simulink model "TSR_System"  (Simulink 7.8)
settings: Solver=ode5  StartTime=0.0  StopTime=inf  FixedStep=1/100  RelTol=1e-3
undefined symbols (not defined in the file): gray, Rec, SDTV
libraries: simulink x4, visionanalysis x2, visiontextngfix x2, visionsinks x2, visionconversions x1, visionstatistics x1
settings Model: Creator=Krzysztof  LastModifiedBy=MarcinB
settings OptimizationCC: InlineParams=on
settings DebuggingCC: SolverPrmCheckMsg=none  MultiTaskCondExecSysMsg=none  MultiTaskRateTransMsg=warning  FcnCallInpInsideContextMsg=Use local settings
settings SFSimCC: SimParseCustomCode=off

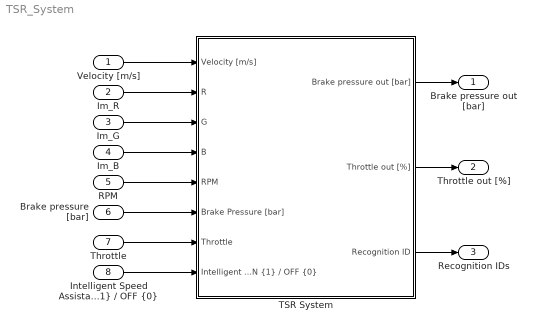
== system TSR_System ==
  Velocity [m/s] : Inport  Interpolate=off
  Im_R : Inport  Port=2
  Im_G : Inport  Port=3
  Im_B : Inport  Port=4
  RPM : Inport  Port=5
  Brake pressure [bar] : Inport  Port=6
  Throttle : Inport  Port=7
  "Intelligent Speed Assistance ON {1} / OFF {0}" : Inport  Port=8
  TSR System : Subsystem  mask{exp_freq=25, dfreq=50, GUI_freq=25, ImgRes=[600 800], DetectionTreshholdValue=0.75, RecognitionTreshholdValue=0.75, NumLimit=5, cdt=3, gdt=5, Tblink=0.5, MaxBrakePressure=150, Perc=20}
      mask prompts: exp_freq "Experiments frequency [Hz]"; dfreq "System frequency [Hz]"; GUI_freq "GUI display frequency [Hz]"; ImgRes "Image resolution"; DetectionTreshholdValue "Detection treshhold value"; RecognitionTreshholdValue "Recognition treshhold value"; NumLimit "Maximum number of objects to extract from image"; cdt "Holding time of recognized sign (colour) [s]"; gdt "Holding time of recognized sign (gray) [s]"; Tblink "Speed limit warning - blinking period [s]"; MaxBrakePressure "Maximum braking pressure [bar]"; Perc "Maximum applicable percentage of deceleration by ISA [%]"
      mask init:
      | %% Generate templates (mat files) if missing
      | if ~exist('DetectTemplates.mat','file')
      |     detection_templates;
      | end
      | if ~exist('RecognitionTemplates.mat','file')
      |     recognition_templates;
      | end
      | 
      | % Load templates into workspace
      | load DetectTemplates.mat
      | load RecognitionTemplates.mat
      | 
      | % Number of templates
      | NoD = size(DetectTemplates,2);
      | NoR = size(RecognitionTemplates,2);
  Brake pressure out [bar] : Outport
  Throttle out [%] : Outport  Port=2
  Recognition IDs : Outport  Port=3
  wires:
  Im_R/1 -> TSR System/2(R)
  Im_G/1 -> TSR System/3(G)
  Im_B/1 -> TSR System/4(B)
  Velocity [m/s]/1 -> TSR System/1(Velocity [m/s])
  Brake pressure [bar]/1 -> TSR System/6(Brake Pressure [bar])
  RPM/1 -> TSR System/5(RPM)
  TSR System/1(Brake pressure out [bar]) -> Brake pressure out [bar]/1
  "Intelligent Speed Assistance ON {1} / OFF {0}"/1 -> TSR System/8("Intelligent Speed Assistance ON {1} / OFF {0}")
  Throttle/1 -> TSR System/7(Throttle)
  TSR System/2("Throttle out [%] ") -> Throttle out [%]/1
  TSR System/3(Recognition ID) -> Recognition IDs/1

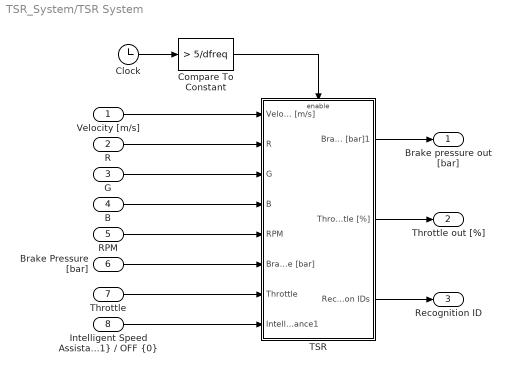
== system TSR_System/TSR System ==
  Velocity [m/s] : Inport  SampleTime=[0 0]
  R : Inport  Port=2  OutDataTypeStr=uint8  PortDimensions=ImgRes
  G : Inport  Port=3  OutDataTypeStr=uint8  PortDimensions=ImgRes
  B : Inport  Port=4  OutDataTypeStr=uint8  PortDimensions=ImgRes
  RPM : Inport  Port=5  SampleTime=[0 0]
  Brake Pressure [bar] : Inport  Port=6  SampleTime=[0 0]
  Throttle : Inport  Port=7
  "Intelligent Speed Assistance ON {1} / OFF {0}" : Inport  Port=8
  Clock : Clock
  Compare To Constant : simulink/Logic and Bit Operations/Compare To Constant  relop=>  const=5/dfreq  OutDataTypeStr=boolean
  TSR : Subsystem
  Brake pressure out [bar] : Outport
  "Throttle out [%] " : Outport  Port=2
  Recognition ID : Outport  Port=3
  wires:
  Clock/1 -> Compare To Constant/1
  Compare To Constant/1 -> TSR/Enable
  TSR/1(Braking pressure [bar]1) -> Brake pressure out [bar]/1
  TSR/2(Throttle [%]) -> "Throttle out [%] "/1
  TSR/3(Recognition IDs) -> Recognition ID/1
  Velocity [m/s]/1 -> TSR/1(Velocity [m/s])
  R/1 -> TSR/2(R)
  G/1 -> TSR/3(G)
  B/1 -> TSR/4(B)
  RPM/1 -> TSR/5(RPM)
  Throttle/1 -> TSR/7(Throttle)
  "Intelligent Speed Assistance ON {1} / OFF {0}"/1 -> TSR/8(Intelligent Speed Assistance1)
  Brake Pressure [bar]/1 -> TSR/6(Brake Pressure [bar])

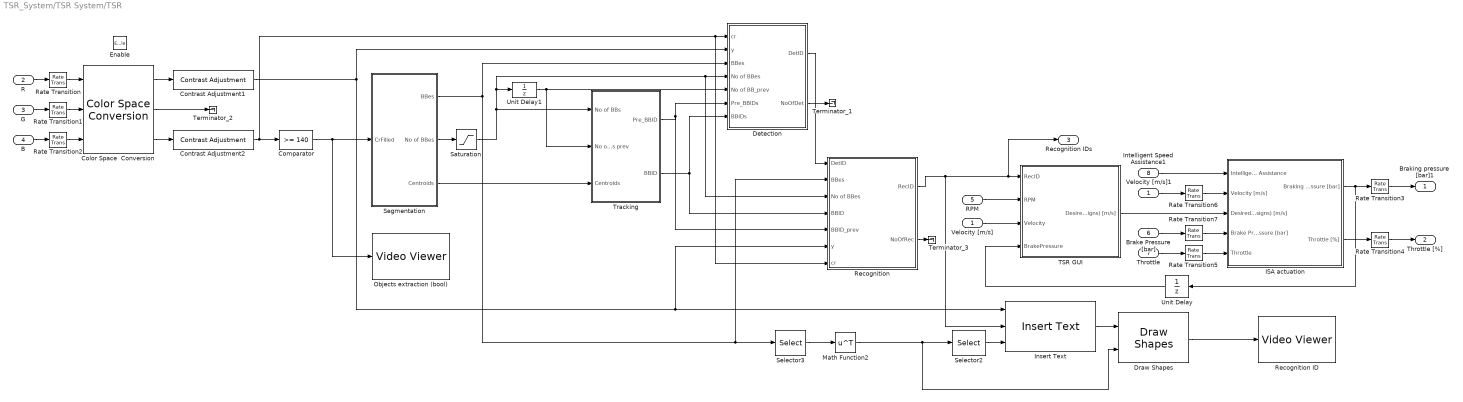
== system TSR_System/TSR System/TSR ==
  Velocity [m/s] : Inport  SampleTime=[0 0]
  R : Inport  Port=2  OutDataTypeStr=uint8  PortDimensions=ImgRes
  G : Inport  Port=3
  B : Inport  Port=4  OutDataTypeStr=uint8  PortDimensions=ImgRes
  RPM : Inport  Port=5  SampleTime=[0 0]
  Brake Pressure [bar] : Inport  Port=6  SampleTime=[0 0]
  Throttle : Inport  Port=7  SampleTime=0
  Intelligent Speed Assistance1 : Inport  Port=8
  Enable : EnablePort
  Color Space  Conversion : visionconversions/Color Space  Conversion  conversion=Obsolete  conversionActive=R'G'B' to Y'CbCr  wp_str=D65  rec=Rec. 601 (SDTV)  sys=1125/60/2:1  imagePorts=Separate color signals
  Comparator : simulink/Logic and Bit Operations/Compare To Constant  relop=>=  const=140  OutDataTypeStr=boolean
  Contrast Adjustment1 : visionanalysis/Contrast Adjustment  methodInputRange=Full input data range [min max]  rangeIn=[0 255]  fracSaturate=[1 1]  isBinNum=on  binNum=256  methodOutputRange=Full data type range  rangeOut=[0 255]  prod1Mode=Binary point scaling  prod1WordLength=32  prod1FracLength=16  prod2Mode=Binary point scaling  prod2WordLength=32  prod2FracLength=16  roundingMode=Floor  overflowMode=off
  Contrast Adjustment2 : visionanalysis/Contrast Adjustment  methodInputRange=Full input data range [min max]  rangeIn=[0 255]  fracSaturate=[1 1]  isBinNum=on  binNum=256  methodOutputRange=Full data type range  rangeOut=[0 255]  prod1Mode=Binary point scaling  prod1WordLength=32  prod1FracLength=16  prod2Mode=Binary point scaling  prod2WordLength=32  prod2FracLength=16  roundingMode=Floor  overflowMode=off
  Detection : Subsystem
  Draw Shapes : visiontextngfix/Draw Shapes  shape=Rectangles  fill=off  fillClrSource=Specify via dialog  display=White  intensity=200  color=[200 255 100]  opacity=0.6  viewport=Entire image  antialiasing=off  inType=Obsolete  imagePorts=One multidimensional signal  prodOutputMode=Binary point scaling  prodOutputWordLength=32  prodOutputFracLength=14  memoryMode=Specify word length  memoryWordLength=16  memoryFracLength=15  roundingMode=Floor  overflowMode=off
  ISA actuation : Subsystem
  Insert Text : visiontextngfix/Insert Text  inputType=Obsolete  theText='%d'  fontFace=LucidaSansRegular  dummyVar1=0  blockFontSize=12  antiAliased=on  getTextLocFrom=Input port  textLoc=[1 1]  getTextColorFrom=Specify via dialog  textColor=255*ones(1,NumLimit);  getTextIntensityFrom=Specify via dialog  textIntensity=0  getTextOpacityFrom=Specify via dialog  textOpacity=1.0  dummyVar2=0  dummyVar3=0  dummyVar4=0  imagePorts=One multidimensional signal  isInputTransposed=off
  Math Function2 : Math  Operator=transpose  SaturateOnIntegerOverflow=on
  Objects extraction (bool) : visionsinks/Video Viewer  inputType=Obsolete7b  imagePorts=One multidimensional signal  useColorMap=off  colormapValue=gray(256)  specRange=off  minInputVal=0  maxInputVal=255  FigPos=[1027 701 606 494]  AxisZoom=on  trueSizedOnce=off  OpenAtMdlStart=on
  Rate Transition : RateTransition  Integrity=off  OutPortSampleTime=1/dfreq
  Rate Transition1 : RateTransition  Integrity=off  OutPortSampleTime=1/dfreq
  Rate Transition2 : RateTransition  Integrity=off  OutPortSampleTime=1/dfreq
  Rate Transition3 : RateTransition  Integrity=off  OutPortSampleTime=0
  Rate Transition4 : RateTransition  Integrity=off  OutPortSampleTime=0
  Rate Transition5 : RateTransition  Integrity=off  OutPortSampleTime=1/GUI_freq
  Rate Transition6 : RateTransition  Integrity=off  OutPortSampleTime=1/GUI_freq
  Rate Transition7 : RateTransition  Integrity=off  OutPortSampleTime=1/GUI_freq
  Recognition : Subsystem
  Recognition ID : visionsinks/Video Viewer  inputType=Obsolete7b  imagePorts=One multidimensional signal  useColorMap=off  colormapValue=gray(256)  specRange=off  minInputVal=0  maxInputVal=255  FigPos=[130 747 808 632]  AxisZoom=on  trueSizedOnce=off  OpenAtMdlStart=on
  Saturation : Saturate  UpperLimit=NumLimit  LowerLimit=0
  Segmentation : Subsystem
  Selector2 : Selector  NumberOfDimensions=2  InputPortWidth=3  IndexOptions=Select all,Index vector (dialog)  Indices=[1 2],[1, 2]  OutputSizes=1,1
  Selector3 : Selector  NumberOfDimensions=2  InputPortWidth=3  IndexOptions=Index vector (dialog),Select all  Indices=[2, 1, 4, 3],1  OutputSizes=1,1
  TSR GUI : Subsystem
  Terminator_1 : Terminator
  Terminator_2 : Terminator
  Terminator_3 : Terminator
  Tracking : Subsystem
  Unit Delay : UnitDelay  SampleTime=-1
  Unit Delay1 : UnitDelay  SampleTime=-1
  Velocity [m/s]1 : InportShadow  Port=1  SampleTime=[0 0]
  Braking pressure [bar]1 : Outport
  Throttle [%] : Outport  Port=2
  Recognition IDs : Outport  Port=3  SampleTime=1/dfreq
  wires:
  Color Space  Conversion/3 -> Contrast Adjustment2/1
  Color Space  Conversion/1 -> Contrast Adjustment1/1
  Color Space  Conversion/2 -> Terminator_2/1
  Segmentation/1(BBes) -> Detection/3(BBes), Recognition/2(BBes), Selector3/1
  Segmentation/2(No of BBes) -> Saturation/1
  Contrast Adjustment2/1 -> Comparator/1, Detection/1(cr), Recognition/7(cr)
  Segmentation/3(Centroids) -> Tracking/3(Centroids)
  Tracking/2(BBID) -> Detection/7(BBIDs), Recognition/4(BBID)
  Tracking/1(Pre_BBID) -> Detection/6(Pre_BBIDs), Recognition/5(BBID_prev)
  Contrast Adjustment1/1 -> Detection/2(y), Recognition/6(y), Insert Text/1
  Unit Delay1/1 -> Tracking/2(No of BBs prev), Detection/5(No of BB_prev)
  Recognition/1(RecID) -> TSR GUI/1(RecID), Recognition IDs/1, Insert Text/2
  R/1 -> Rate Transition/1
  G/1 -> Rate Transition1/1
  B/1 -> Rate Transition2/1
  Rate Transition/1 -> Color Space  Conversion/1
  Rate Transition1/1 -> Color Space  Conversion/2
  Rate Transition2/1 -> Color Space  Conversion/3
  Saturation/1 -> Unit Delay1/1, Detection/4(No of BBes), Recognition/3(No of BBes), Tracking/1(No of BBs)
  Velocity [m/s]/1 -> TSR GUI/3(Velocity)
  RPM/1 -> TSR GUI/2(RPM)
  Unit Delay/1 -> TSR GUI/4(BrakePressure)
  Throttle/1 -> Rate Transition5/1
  ISA actuation/1(Braking pressure [bar]) -> Unit Delay/1, Rate Transition3/1
  ISA actuation/2(Throttle [%]) -> Rate Transition4/1
  Velocity [m/s]1/1 -> Rate Transition6/1
  Brake Pressure [bar]/1 -> Rate Transition7/1
  Rate Transition7/1 -> ISA actuation/4(Brake Pressure [bar])
  Rate Transition3/1 -> Braking pressure [bar]1/1
  Rate Transition4/1 -> Throttle [%]/1
  Rate Transition5/1 -> ISA actuation/5(Throttle)
  Intelligent Speed Assistance1/1 -> ISA actuation/1(Intelligent Speed  Assistance)
  Rate Transition6/1 -> ISA actuation/2(Velocity [m/s])
  TSR GUI/1(Desired vel (signs) [m/s]) -> ISA actuation/3(Desired vel (signs) [m/s])
  Detection/1(DetID) -> Recognition/1(DetID)
  Detection/2(NoOfDet) -> Terminator_1/1
  Comparator/1 -> Segmentation/1(CrFilled), Objects extraction (bool)/1
  Recognition/2(NoOfRec) -> Terminator_3/1
  Insert Text/1 -> Draw Shapes/1
  Selector2/1 -> Insert Text/3
  Selector3/1 -> Math Function2/1
  Math Function2/1 -> Draw Shapes/2, Selector2/1
  Draw Shapes/1 -> Recognition ID/1

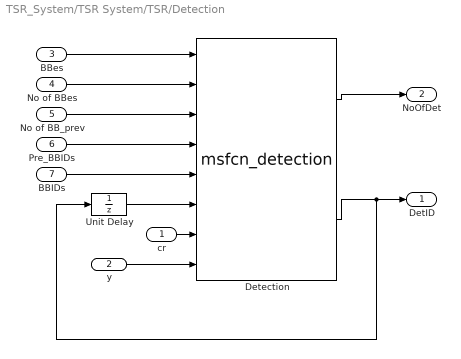
== system TSR_System/TSR System/TSR/Detection ==
  cr : Inport
  y : Inport  Port=2
  BBes : Inport  Port=3
  No of BBes : Inport  Port=4
  No of BB_prev : Inport  Port=5
  Pre_BBIDs : Inport  Port=6
  BBIDs : Inport  Port=7
  Detection : M-S-Function  FunctionName=msfcn_detection  Parameters=DetectTemplates, NoD, ImgRes, NumLimit, DetectionTreshholdValue
      mask Display:
      | port_label('input', 1, 'BBes');
      | port_label('input', 2, 'NoBB');
      | port_label('input', 3, 'NoBBp');
      | port_label('input', 4, 'Pre_BBID');
      | port_label('input', 5, 'BBID');
      | port_label('input', 6, 'Pre_DetID');
      | port_label('input', 7, 'cr');
      | port_label('input', 8, 'y');
      | 
      | port_label('output', 1, 'No of detections');
      | port_label('output', 2, 'DetID');
  Unit Delay : UnitDelay  X0=zeros(NumLimit,1);  SampleTime=-1
  DetID : Outport
  NoOfDet : Outport  Port=2
  wires:
  Detection/1 -> NoOfDet/1
  Detection/2 -> DetID/1, Unit Delay/1
  BBes/1 -> Detection/1
  No of BBes/1 -> Detection/2
  No of BB_prev/1 -> Detection/3
  Pre_BBIDs/1 -> Detection/4
  BBIDs/1 -> Detection/5
  Unit Delay/1 -> Detection/6
  cr/1 -> Detection/7
  y/1 -> Detection/8

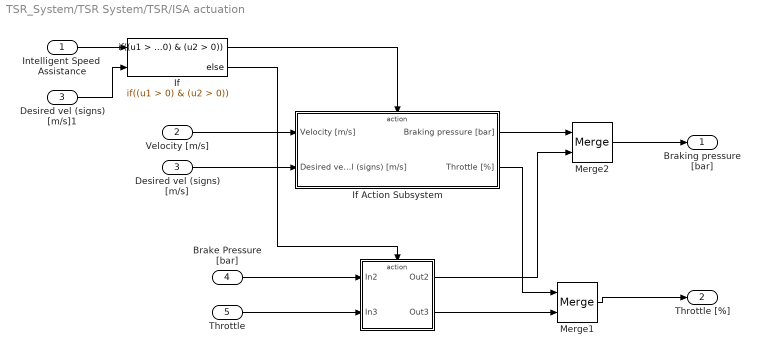
== system TSR_System/TSR System/TSR/ISA actuation ==
  Intelligent Speed  Assistance : Inport
  Velocity [m/s] : Inport  Port=2
  Desired vel (signs) [m/s] : Inport  Port=3
  Brake Pressure [bar] : Inport  Port=4
  Throttle : Inport  Port=5
  " " : Subsystem  TreatAsAtomicUnit=on
  Desired vel (signs) [m/s]1 : InportShadow  Port=3
  If : If  NumInputs=2  IfExpression=(u1 > 0) & (u2 > 0)
  If Action Subsystem : Subsystem  TreatAsAtomicUnit=on
  Merge1 : Merge  InitialOutput=0
  Merge2 : Merge  InitialOutput=0
  Braking pressure [bar] : Outport
  Throttle [%] : Outport  Port=2
  wires:
  Intelligent Speed  Assistance/1 -> If/1
  If/1 -> If Action Subsystem/Action
  Brake Pressure [bar]/1 -> " "/1(In2)
  Throttle/1 -> " "/2(In3)
  " "/2(Out3) -> Merge1/2
  Merge1/1 -> Throttle [%]/1
  Merge2/1 -> Braking pressure [bar]/1
  If Action Subsystem/2(Throttle [%]) -> Merge1/1
  " "/1(Out2) -> Merge2/2
  If Action Subsystem/1(Braking pressure [bar]) -> Merge2/1
  Desired vel (signs) [m/s]/1 -> If Action Subsystem/2(Desired vel (signs) [m/s])
  Velocity [m/s]/1 -> If Action Subsystem/1(Velocity [m/s])
  Desired vel (signs) [m/s]1/1 -> If/2
  If/2 -> " "/Action

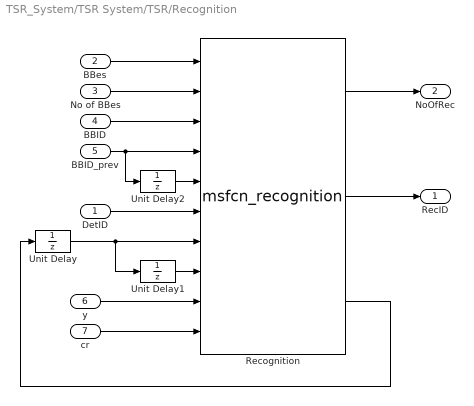
== system TSR_System/TSR System/TSR/Recognition ==
  DetID : Inport
  BBes : Inport  Port=2
  No of BBes : Inport  Port=3
  BBID : Inport  Port=4
  BBID_prev : Inport  Port=5
  y : Inport  Port=6
  cr : Inport  Port=7
  Recognition : M-S-Function  FunctionName=msfcn_recognition  Parameters=RecognitionTemplates, NoR, ImgRes, NumLimit, RecognitionTreshholdValue
      mask Display:
      | port_label('input', 1, 'BBes');
      | port_label('input', 2, 'NoBB');
      | port_label('input', 3, 'BBID');
      | port_label('input', 4, 'BBIDp');
      | port_label('input', 5, 'BBIDpp');
      | port_label('input', 6, 'DetID');
      | port_label('input', 7, 'RecIDp');
      | port_label('input', 8, 'RecIDpp');
      | port_label('input', 9, 'y');
      | port_label('input',10, 'cr');
      | 
      | 
      | port_label('output', 1, 'No of recognitions');
      | port_label('output', 2, 'RecIDfinal');
      | port_label('output', 3, 'RecID');
  Unit Delay : UnitDelay  X0=zeros(NumLimit,1);  SampleTime=-1
  Unit Delay1 : UnitDelay  X0=zeros(NumLimit,1);  SampleTime=-1
  Unit Delay2 : UnitDelay  X0=zeros(NumLimit,1);  SampleTime=-1
  RecID : Outport
  NoOfRec : Outport  Port=2
  wires:
  Recognition/1 -> NoOfRec/1
  BBID_prev/1 -> Unit Delay2/1, Recognition/4
  Recognition/3 -> Unit Delay/1
  Recognition/2 -> RecID/1
  BBes/1 -> Recognition/1
  No of BBes/1 -> Recognition/2
  BBID/1 -> Recognition/3
  Unit Delay2/1 -> Recognition/5
  DetID/1 -> Recognition/6
  Unit Delay/1 -> Recognition/7, Unit Delay1/1
  Unit Delay1/1 -> Recognition/8
  y/1 -> Recognition/9
  cr/1 -> Recognition/10

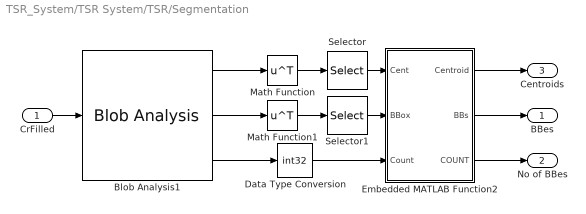
== system TSR_System/TSR System/TSR/Segmentation ==
  CrFilled : Inport
  Blob Analysis1 : visionstatistics/Blob Analysis  Tag=vipblks_row_conv  area=off  centroid=on  bBox=on  majorAxis=off  minorAxis=off  angle=off  eccentricity=off  equivDiameterSq=off  extent=off  perimeter=off  maxBlobs=NumLimit  warnIfNumBlobsExceeded=off  isCount=on  useMinArea=on  minArea=16*16  useMaxArea=on  maxArea=0.02*ImgRes(1)*ImgRes(2)  excludeBorderBlob=on  outDT=double  isOutVarDim=off  isFill=on  fillValues=0  conn=8  isLabel=off  outputMode=Binary point scaling  outputWordLength=32  outputFracLength=16  firstCoeffMode=Binary point scaling  firstCoeffWordLength=16  firstCoeffFracLength=14  secondCoeffMode=Binary point scaling  secondCoeffWordLength=32  secondCoeffFracLength=16  accumMode=Binary point scaling  accumWordLength=32  accumFracLength=0  prodOutputMode=Binary point scaling  prodOutputWordLength=32  prodOutputFracLength=16  roundingMode=Floor  overflowMode=off
  Data Type Conversion : DataTypeConversion  OutDataTypeStr=int32
  Embedded MATLAB Function2 : MATLAB Function  TreatAsAtomicUnit=on
  Math Function : Math  Operator=transpose  SaturateOnIntegerOverflow=on
  Math Function1 : Math  Operator=transpose  SaturateOnIntegerOverflow=on
  Selector : Selector  NumberOfDimensions=2  InputPortWidth=2  IndexOptions=Index vector (dialog),Select all  Indices=[2 1],1  OutputSizes=1,1
  Selector1 : Selector  NumberOfDimensions=2  InputPortWidth=2  IndexOptions=Index vector (dialog),Select all  Indices=[2 1 4 3],  OutputSizes=1,1
  BBes : Outport
  No of BBes : Outport  Port=2
  Centroids : Outport  Port=3
  wires:
  CrFilled/1 -> Blob Analysis1/1
  Blob Analysis1/3 -> Data Type Conversion/1
  Data Type Conversion/1 -> Embedded MATLAB Function2/3(Count)
  Embedded MATLAB Function2/1(Centroid) -> Centroids/1
  Embedded MATLAB Function2/2(BBs) -> BBes/1
  Embedded MATLAB Function2/3(COUNT) -> No of BBes/1
  Blob Analysis1/1 -> Math Function/1
  Math Function/1 -> Selector/1
  Blob Analysis1/2 -> Math Function1/1
  Math Function1/1 -> Selector1/1
  Selector/1 -> Embedded MATLAB Function2/1(Cent)
  Selector1/1 -> Embedded MATLAB Function2/2(BBox)

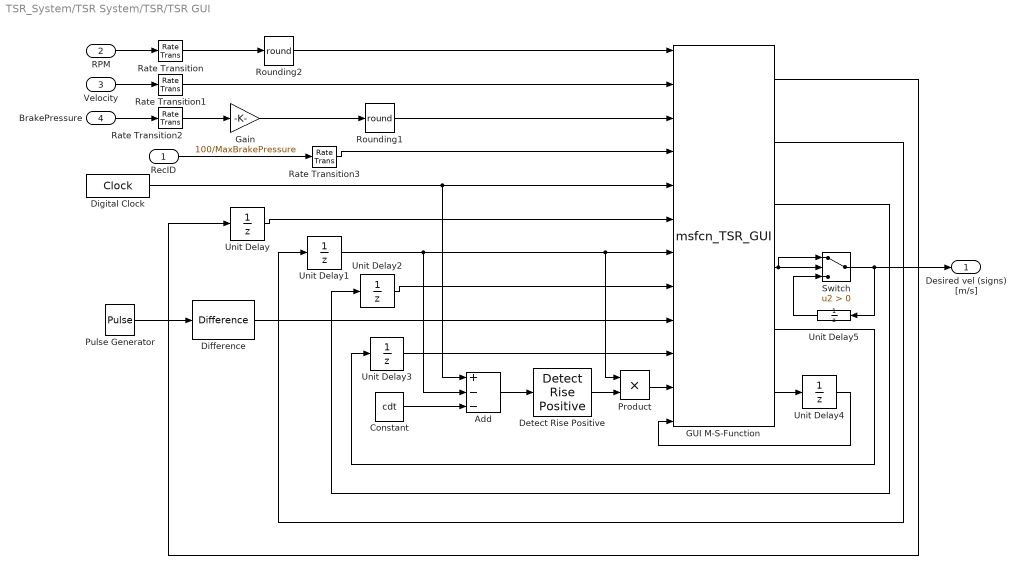
== system TSR_System/TSR System/TSR/TSR GUI ==
  RecID : Inport
  RPM : Inport  Port=2
  Velocity : Inport  Port=3
  BrakePressure : Inport  Port=4
  Add : Sum  Inputs=+--
  Constant : Constant  Value=cdt
  Detect Rise Positive : simulink/Logic and Bit Operations/Detect Rise Positive  vinit=0  InputProcessing=Inherited  OutDataTypeStr=uint8
  Difference : simulink/Discrete/Difference  ICPrevInput=0.0  InputProcessing=Inherited  OutMin=[]  OutMax=[]  OutDataType=fixdt(1, 16)  OutScaling=2^-10  DoSatur=off
  Digital Clock : DigitalClock  SampleTime=1/GUI_freq
  GUI M-S-Function : M-S-Function  FunctionName=msfcn_TSR_GUI  Parameters=GUI_freq, RecognitionTemplates, cdt, gdt, NumLimit
      mask Display:
      | port_label('input',1,'RPM');
      | port_label('input',2,'V');
      | port_label('input',3,'BrakePress');
      | port_label('input',4,'RecID');
      | port_label('input',5,'Clock');
      | port_label('input',6,'Slots IDs prev');
      | port_label('input',7,'Slots t prev');
      | port_label('input',8,'Slots DesVel prev');
      | port_label('input',9,'Impulse gen');
      | port_label('input',10,'Warn prev');
      | port_label('input',11,'Display trigger');
      | port_label('input',12,'Slots gray prev');
      | 
      | port_label('output',1,'Slots (ID)');
      | port_label('output',2,'Slots (time)');
      | port_label('output',3,'Slots (DesVel)');
      | port_label('output',4,'Desired velocity (signs) [m/s]');
      | port_label('output',5,'Warning');
      | port_label('output',6,'Slots (gray)');
  Gain : Gain  Gain=100/MaxBrakePressure
  Product : Product  RndMeth=Zero
  Pulse Generator : DiscretePulseGenerator  Period=round ( Tblink * GUI_freq )  PulseWidth=round ( 0.5 * Tblink * GUI_freq )  PhaseDelay=round ( 0.25 * Tblink * GUI_freq )  SampleTime=1/GUI_freq
  Rate Transition{,1..3} (4 alike) : RateTransition  Integrity=off  OutPortSampleTime=1/GUI_freq
  Rounding1 : Rounding  Operator=round
  Rounding2 : Rounding  Operator=round
  Switch : Switch  Criteria=u2 > Threshold
  Unit Delay : UnitDelay  X0=zeros(3,1,'int32')  SampleTime=-1
  Unit Delay1 : UnitDelay  X0=zeros(3,1,'int32')  SampleTime=-1
  Unit Delay2 : UnitDelay  X0=zeros(3,1)  SampleTime=-1
  Unit Delay3 : UnitDelay  X0=false(1)  SampleTime=-1
  Unit Delay4 : UnitDelay  X0=false(1)  SampleTime=-1
  Unit Delay5 : UnitDelay  SampleTime=-1
  Desired vel (signs) [m/s] : Outport  SampleTime=1/GUI_freq
  wires:
  RPM/1 -> Rate Transition/1
  Velocity/1 -> Rate Transition1/1
  BrakePressure/1 -> Rate Transition2/1
  Digital Clock/1 -> GUI M-S-Function/5, Add/1
  Unit Delay/1 -> GUI M-S-Function/6
  GUI M-S-Function/1 -> Unit Delay/1
  RecID/1 -> Rate Transition3/1
  Unit Delay1/1 -> GUI M-S-Function/7, Product/1, Add/2
  GUI M-S-Function/2 -> Unit Delay1/1
  Gain/1 -> Rounding1/1
  Rounding1/1 -> GUI M-S-Function/3
  Rate Transition/1 -> Rounding2/1
  Rate Transition1/1 -> GUI M-S-Function/2
  Rate Transition2/1 -> Gain/1
  Rounding2/1 -> GUI M-S-Function/1
  Unit Delay2/1 -> GUI M-S-Function/8
  GUI M-S-Function/3 -> Unit Delay2/1
  Difference/1 -> GUI M-S-Function/9
  Pulse Generator/1 -> Difference/1
  Rate Transition3/1 -> GUI M-S-Function/4
  Unit Delay3/1 -> GUI M-S-Function/10
  GUI M-S-Function/5 -> Unit Delay3/1
  Add/1 -> Detect Rise Positive/1
  Constant/1 -> Add/3
  Product/1 -> GUI M-S-Function/11
  Detect Rise Positive/1 -> Product/2
  GUI M-S-Function/6 -> Unit Delay4/1
  Unit Delay4/1 -> GUI M-S-Function/12
  GUI M-S-Function/4 -> Switch/2, Switch/1
  Switch/1 -> Desired vel (signs) [m/s]/1, Unit Delay5/1
  Unit Delay5/1 -> Switch/3

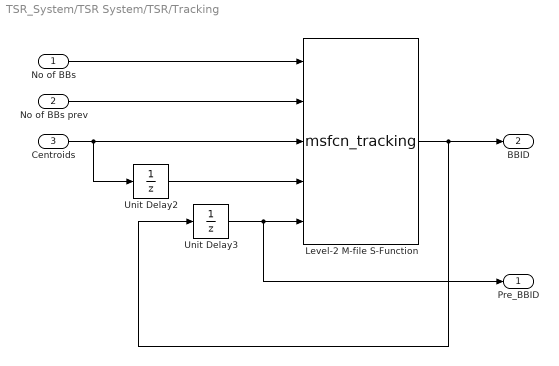
== system TSR_System/TSR System/TSR/Tracking ==
  No of BBs : Inport
  No of BBs prev : Inport  Port=2
  Centroids : Inport  Port=3
  Level-2 M-file S-Function : M-S-Function  FunctionName=msfcn_tracking  Parameters=NumLimit
      mask Display:
      | port_label('input', 1, 'NoBB');
      | port_label('input', 2, 'NoBBp');
      | port_label('input', 3, 'Centr');
      | port_label('input', 4, 'CentrP');
      | port_label('input', 5, 'BBIDp');
      | port_label('output',1, 'BBIDn');
  Unit Delay2 : UnitDelay  X0=zeros(2,NumLimit)  SampleTime=-1
  Unit Delay3 : UnitDelay  X0=zeros(NumLimit,1)  SampleTime=-1
  Pre_BBID : Outport
  BBID : Outport  Port=2
  wires:
  No of BBs/1 -> Level-2 M-file S-Function/1
  Centroids/1 -> Unit Delay2/1, Level-2 M-file S-Function/3
  Level-2 M-file S-Function/1 -> Unit Delay3/1, BBID/1
  No of BBs prev/1 -> Level-2 M-file S-Function/2
  Unit Delay2/1 -> Level-2 M-file S-Function/4
  Unit Delay3/1 -> Level-2 M-file S-Function/5, Pre_BBID/1

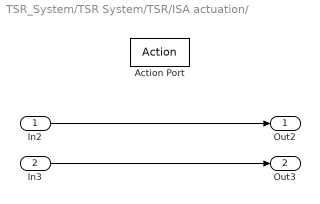
== system TSR_System/TSR System/TSR/ISA actuation/  ==
  In2 : Inport
  In3 : Inport  Port=2
  Action Port : ActionPort  ActionType=else
  Out2 : Outport  InitialOutput=0
  Out3 : Outport  Port=2  InitialOutput=0
  wires:
  In2/1 -> Out2/1
  In3/1 -> Out3/1

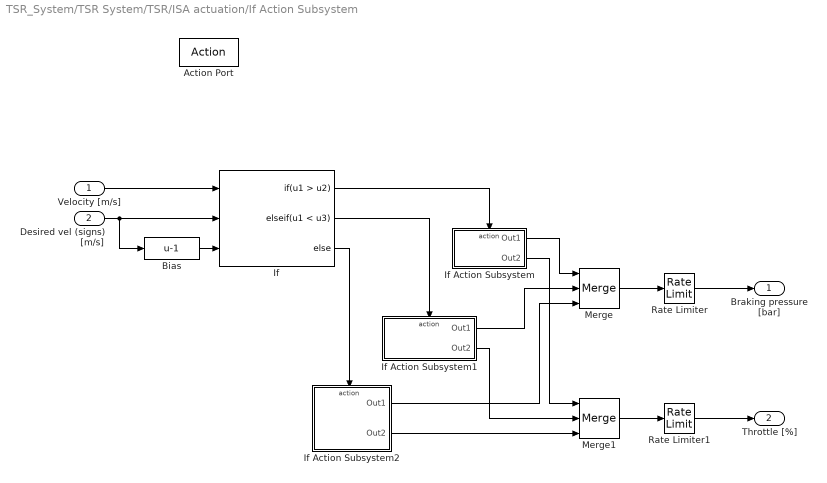
== system TSR_System/TSR System/TSR/ISA actuation/If Action Subsystem ==
  Velocity [m/s] : Inport
  Desired vel (signs) [m/s] : Inport  Port=2
  Action Port : ActionPort  ActionType=then
  Bias : Bias  Bias=-1
  If : If  NumInputs=3  IfExpression=u1 > u2  ElseIfExpressions=u1 < u3
  If Action Subsystem : Subsystem  TreatAsAtomicUnit=on
  If Action Subsystem1 : Subsystem  TreatAsAtomicUnit=on
  If Action Subsystem2 : Subsystem  TreatAsAtomicUnit=on
  Merge : Merge  Inputs=3  InitialOutput=0
  Merge1 : Merge  Inputs=3  InitialOutput=0
  Rate Limiter : RateLimiter  RisingSlewLimit=MaxBrakePressure  FallingSlewLimit=-MaxBrakePressure  SampleTimeMode=inherited
  Rate Limiter1 : RateLimiter  RisingSlewLimit=15  FallingSlewLimit=-inf  SampleTimeMode=inherited
  Braking pressure [bar] : Outport  InitialOutput=0
  Throttle [%] : Outport  Port=2  InitialOutput=0
  wires:
  Velocity [m/s]/1 -> If/1
  Desired vel (signs) [m/s]/1 -> If/2, Bias/1
  Bias/1 -> If/3
  If/1 -> If Action Subsystem/Action
  If/2 -> If Action Subsystem1/Action
  If/3 -> If Action Subsystem2/Action
  Merge/1 -> Rate Limiter/1
  Merge1/1 -> Rate Limiter1/1
  Rate Limiter/1 -> Braking pressure [bar]/1
  Rate Limiter1/1 -> Throttle [%]/1
  If Action Subsystem/1(Out1) -> Merge/1
  If Action Subsystem/2(Out2) -> Merge1/1
  If Action Subsystem1/1(Out1) -> Merge/2
  If Action Subsystem1/2(Out2) -> Merge1/2
  If Action Subsystem2/1(Out1) -> Merge/3
  If Action Subsystem2/2(Out2) -> Merge1/3

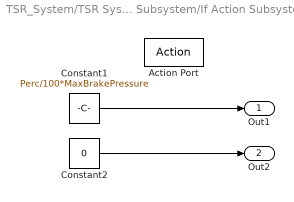
== system TSR_System/TSR System/TSR/ISA actuation/If Action Subsystem/If Action Subsystem ==
  Action Port : ActionPort  ActionType=then
  Constant1 : Constant  Value=Perc/100*MaxBrakePressure
  Constant2 : Constant  Value=0
  Out1 : Outport  InitialOutput=0
  Out2 : Outport  Port=2  InitialOutput=0
  wires:
  Constant1/1 -> Out1/1
  Constant2/1 -> Out2/1

== system TSR_System/TSR System/TSR/ISA actuation/If Action Subsystem/If Action Subsystem1 ==
  Action Port : ActionPort  ActionType=elseif
  Constant1 : Constant  Value=100
  Constant2 : Constant  Value=0
  Out1 : Outport  InitialOutput=0
  Out2 : Outport  Port=2  InitialOutput=0
  wires:
  Constant2/1 -> Out1/1
  Constant1/1 -> Out2/1

== system TSR_System/TSR System/TSR/ISA actuation/If Action Subsystem/If Action Subsystem2 ==
  Action Port : ActionPort  ActionType=else
  Constant1 : Constant  Value=0
  Constant2 : Constant  Value=0
  Out1 : Outport  InitialOutput=0
  Out2 : Outport  Port=2  InitialOutput=0
  wires:
  Constant2/1 -> Out1/1
  Constant1/1 -> Out2/1

== matlab function TSR System/TSR/Segmentation/Embedded MATLAB Function2 ==
  data: Cent input double; Centroid output double; BBox input double; BBs output double; Count input double; COUNT output double; NumLimit parameter double
function [Centroid, BBs, COUNT] = fcn(Cent, BBox, Count, NumLimit)
%#eml

% Output declarations
Centroid = zeros(2,NumLimit);
BBs      = zeros(4,NumLimit,'int32');
COUNT    = zeros(1,'int32');

% Remove non-sign-like BBoxes
coef = 1.5;
scales = zeros(NumLimit,1);
scales(1:Count) = double(BBox(3,1:Count))./double(BBox(4,1:Count));

for ii = 1 : Count
    if ( scales(ii) <= coef ) && ( scales(ii) >= 1/coef)
        COUNT = COUNT + 1;
        BBs(:,COUNT) = BBox(:,ii);
        Centroid(:,COUNT) = Cent(:,ii);
    end
end

end
